simulink model "EX4_Lab02_Group02"  (R2025b)
settings: Solver=VariableStepAuto  StartTime=0.0  StopTime=10  RelTol=1e-3
settings Model: Creator=ASUS  LastModifiedBy=ASUS

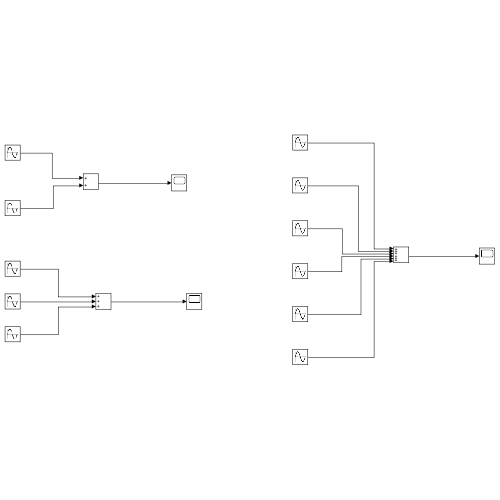
[thumbnail: Simulink's stored preview of the top-level diagram]
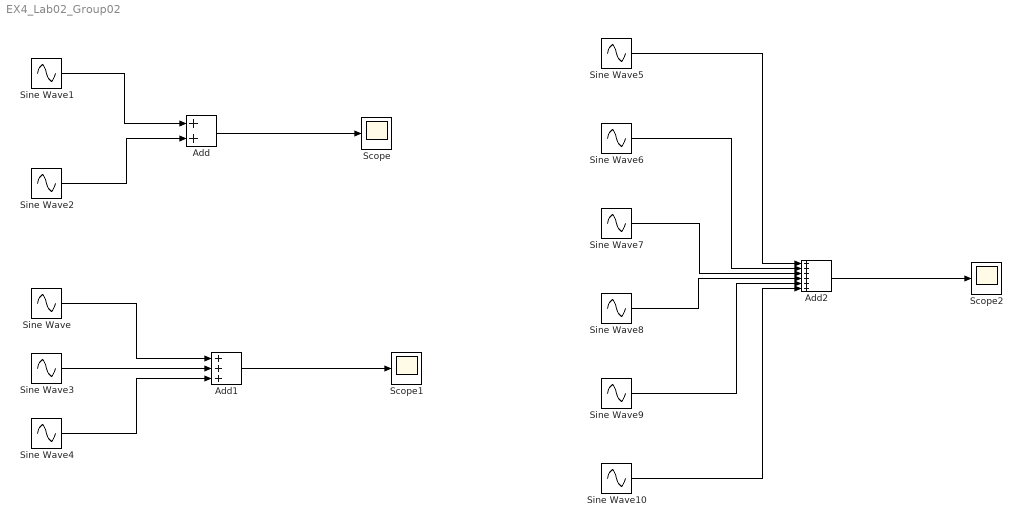
== system EX4_Lab02_Group02 ==
  Add : Sum
  Add1 : Sum  Inputs=+++
  Add2 : Sum  Inputs=++++++
  Scope : Scope
      settings: ActiveDisplayYMinimum=-1.1767968086949239  ActiveDisplayYMaximum=1.1767383715445676
  Scope1 : Scope
      settings: ActiveDisplayYMinimum=-1.140747499756178  ActiveDisplayYMaximum=1.1622900563095389
  Scope2 : Scope
      settings: ActiveDisplayYMinimum=-1.1548630988602879  ActiveDisplayYMaximum=1.1288802884685574  DataLoggingVariableName=ScopeData2
  Sine Wave : Sin  Frequency=2*pi*0.15  SampleTime=0
  Sine Wave1 : Sin  Frequency=2*pi*0.15  SampleTime=0
  Sine Wave10 : Sin  Amplitude=1/11  Frequency=2*pi*11*0.15  SampleTime=0
  Sine Wave2 : Sin  Amplitude=1/3  Frequency=2*pi*0.45  SampleTime=0
  Sine Wave3 : Sin  Amplitude=1/3  Frequency=2*pi*3*0.15  SampleTime=0
  Sine Wave4 : Sin  Amplitude=1/5  Frequency=2*pi*5*0.15  SampleTime=0
  Sine Wave5 : Sin  Frequency=2*pi*0.15  SampleTime=0
  Sine Wave6 : Sin  Amplitude=1/3  Frequency=2*pi*3*0.15  SampleTime=0
  Sine Wave7 : Sin  Amplitude=1/5  Frequency=2*pi*5*0.15  SampleTime=0
  Sine Wave8 : Sin  Amplitude=1/7  Frequency=2*pi*7*0.15  SampleTime=0
  Sine Wave9 : Sin  Amplitude=1/9  Frequency=2*pi*9*0.15  SampleTime=0
  wires:
  Sine Wave1/1 -> Add/1
  Sine Wave2/1 -> Add/2
  Add/1 -> Scope/1
  Sine Wave/1 -> Add1/1
  Sine Wave3/1 -> Add1/2
  Sine Wave4/1 -> Add1/3
  Add1/1 -> Scope1/1
  Sine Wave8/1 -> Add2/4
  Sine Wave5/1 -> Add2/1
  Sine Wave6/1 -> Add2/2
  Sine Wave7/1 -> Add2/3
  Sine Wave9/1 -> Add2/5
  Sine Wave10/1 -> Add2/6
  Add2/1 -> Scope2/1
